simulink model "sim_car_model1"  (R2022a)
settings: Solver=VariableStepAuto  StartTime=0.0  StopTime=500  RelTol=1e-3
values from neighbouring files (symbols this model uses):
  b = (Fmax - c*Vmax^2)/Vmax    (= 2.52478421655)    [Copy_of_script.m]    (also in script.m)
  c = 0.5*rho*A*cd    (= 0.4907934)    [Copy_of_script.m]    (also in script.m)
  g = 9.82    [Copy_of_script.m]    (also in script.m)
  m = 1001    [Copy_of_script.m]    (also in script.m)
settings Model: Creator=gomag  LastModifiedBy=gomag

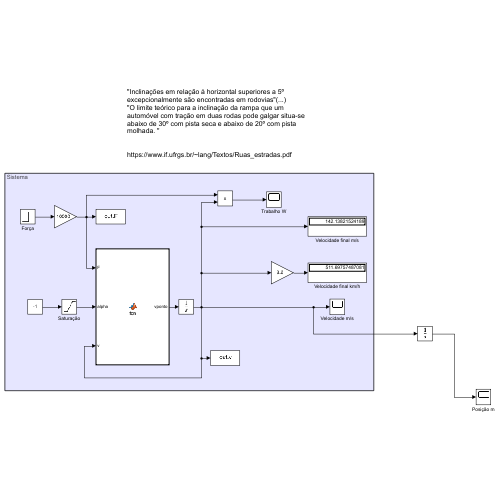
[thumbnail: Simulink's stored preview of the top-level diagram]
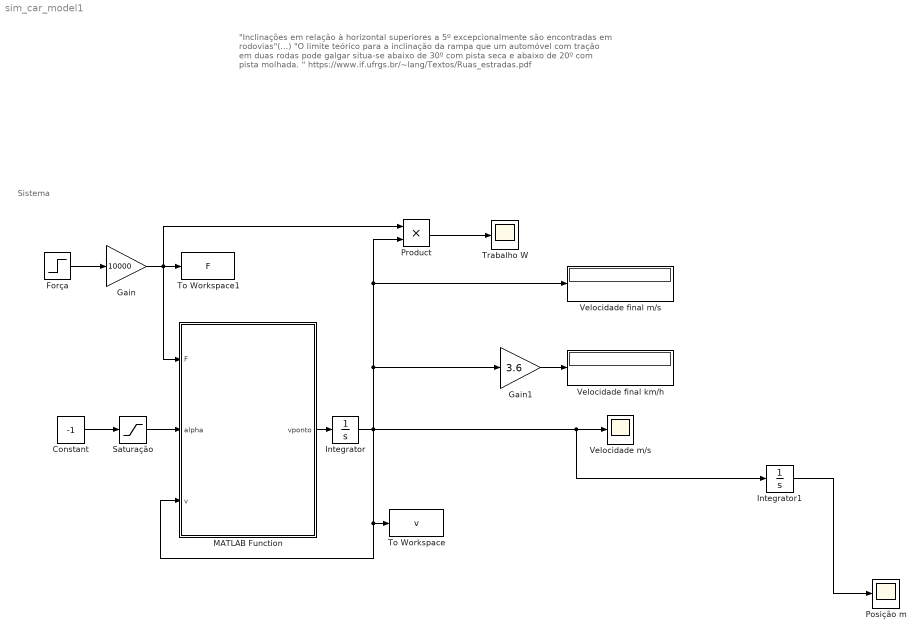
== system sim_car_model1 ==
  note: Sistema
  note: "Inclinações em relação à horizontal superiores a 5º excepcionalmente são encontradas em rodovias"(...)
      | "O limite teórico para a inclinação da rampa que um automóvel com tração em duas rodas pode galgar situa-se abaixo de 30º com pista seca e abaixo de 20º com pista molhada. "
      |
      | https://www.if.ufrgs.br/~lang/Textos/Ruas_estradas.pdf
  Constant : Constant  Value=-1
  Força : Step  SampleTime=0
  Gain : Gain  Gain=10000
  Gain1 : Gain  Gain=3.6
  Integrator : Integrator
  Integrator1 : Integrator
  MATLAB Function : MATLAB Function  TreatAsAtomicUnit=on
  Posição m : Scope
  Product : Product
  Saturação : Saturate  UpperLimit=5/180  LowerLimit=-5/180
  To Workspace : ToWorkspace  VariableName=v  SaveFormat=Timeseries  SampleTime=-1
  To Workspace1 : ToWorkspace  VariableName=F  SaveFormat=Timeseries  SampleTime=-1
  Trabalho W : Scope
  Velocidade final km/h : Display
      settings: Decimation=4
  Velocidade final m/s : Display
      settings: Decimation=4
  Velocidade m/s : Scope
  wires:
  Força/1 -> Gain/1
  Constant/1 -> Saturação/1
  MATLAB Function/1(vponto) -> Integrator/1
  Gain/1 -> Product/1, To Workspace1/1, MATLAB Function/1(F)
  Product/1 -> Trabalho W/1
  Integrator/1 -> Integrator1/1, Velocidade m/s/1, To Workspace/1, MATLAB Function/3(v), Gain1/1, Velocidade final m/s/1, Product/2
  Gain1/1 -> Velocidade final km/h/1
  Integrator1/1 -> Posição m/1
  Saturação/1 -> MATLAB Function/2(alpha)

== matlab function sim_car_model1/MATLAB Function ==
  data: F input; vponto output; alpha input; v input; b parameter; c parameter; m parameter; g parameter
function vponto = fcn(F, alpha, v, b, c, m, g)

vponto=( F - b*v - c*v^2 - m*g*sin(alpha) ) / m;
